simulink library "MyEma"  (R2017a)
settings: Solver=VariableStepAuto  StartTime=0.0  StopTime=10.0  RelTol=1e-3
settings Model: Creator=alexandr.lanin  LastModifiedBy=alexandr.lanin

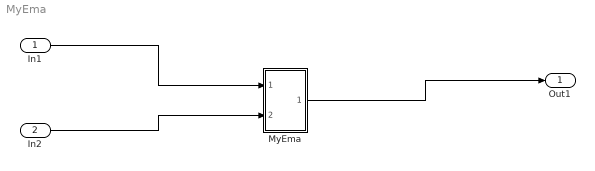
== system MyEma ==
  In1 : Inport
  In2 : Inport  Port=2
  MyEma : Subsystem
  Out1 : Outport
  wires:
  In1/1 -> MyEma/1(In1)
  In2/1 -> MyEma/2(In2)
  MyEma/1(Out1) -> Out1/1

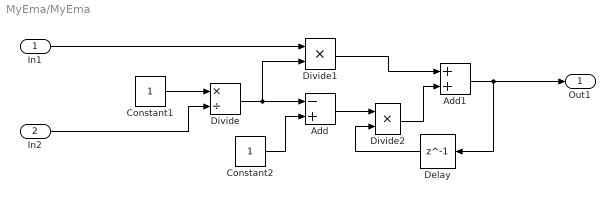
== system MyEma/MyEma ==
  In1 : Inport
  In2 : Inport  Port=2
  Add : Sum  Inputs=-+
  Add1 : Sum
  Constant1 : Constant
  Constant2 : Constant
  Delay : Delay  DelayLength=1  InitialCondition=0
  Divide : Product  Inputs=*/
  Divide1 : Product  Inputs=**
  Divide2 : Product  Inputs=**
  Out1 : Outport
  wires:
  Add1/1 -> Out1/1, Delay/1
  Divide1/1 -> Add1/1
  Divide/1 -> Divide1/2, Add/1
  Delay/1 -> Divide2/2
  Divide2/1 -> Add1/2
  Constant1/1 -> Divide/1
  Add/1 -> Divide2/1
  In1/1 -> Divide1/1
  Constant2/1 -> Add/2
  In2/1 -> Divide/2
